simulink model "ev3_robot_hostcontrol_modified"  (R2019b)
settings: Solver=VariableStepAuto  StartTime=0.0  StopTime=inf  RelTol=1e-3
libraries: instrumentlib x4
settings Model: Creator=The MathWorks, Inc.  LastModifiedBy=Duc
settings DataIOCC: ReturnWorkspaceOutputs=off
settings DebuggingCC: ParameterPrecisionLossMsg=none  ArithmeticOperatorsInVariantConditions=warning
settings SFSimCC: SimUseLocalCustomCode=off  CustomCodeUndefinedFunction=UseInterfaceOnly
settings RTWCC: RTWUseLocalCustomCode=off
settings CodeAppCC: StateflowObjectComments=on

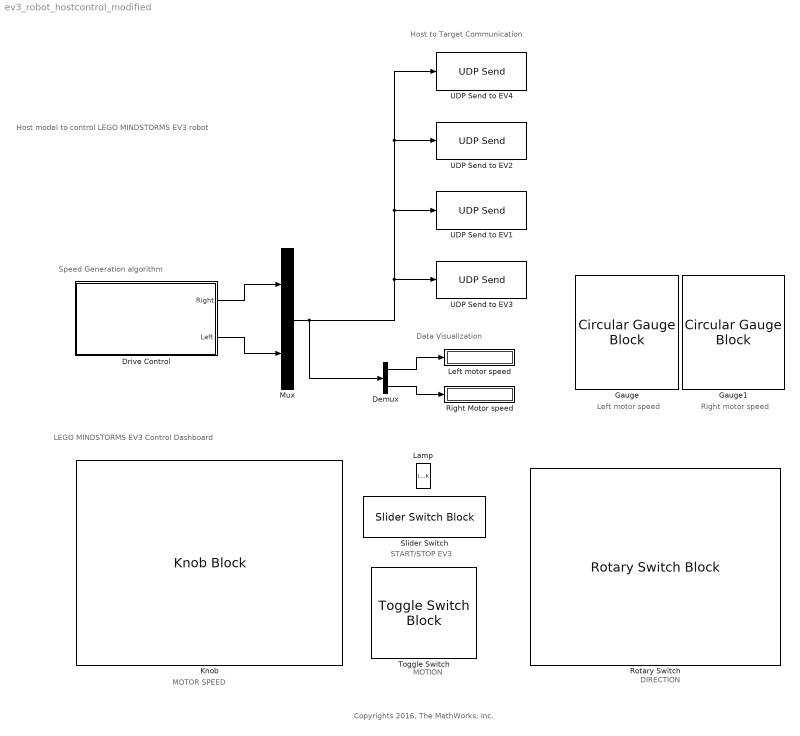
== system ev3_robot_hostcontrol_modified ==
  note: Copyrights 2016, The MathWorks, Inc.
  note: Host model to control
      | LEGO MINDSTORMS EV3 robot
  note: Right motor speed
  note: Left motor speed
  note: DIRECTION
  note: MOTION
  note: START/STOP EV3
  note: MOTOR SPEED
  note: Data Visualization
  note: Host to Target Communication
  note: Speed Generation algorithm
  note: LEGO MINDSTORMS EV3 Control Dashboard
  Demux : Demux  Outputs=2
  Drive Control : Subsystem
  Gauge : CircularGaugeBlock  ScaleMin=-100
  Gauge1 : CircularGaugeBlock  ScaleMin=-100
  Knob : KnobBlock
  Lamp : LampBlock  LabelPosition=Hide
  Left motor speed : Display
  Mux : Mux  Inputs=2
  Right Motor speed : Display
  Rotary Switch : RotarySwitchBlock  LabelPosition=Hide
      settings: Values={{'LEFT', '', 'STRAIGHT', '', 'RIGHT'}, [0 1 2 3 4]}
  Slider Switch : SliderSwitchBlock  LabelPosition=Hide
      settings: Values={{'STOP', 'START'}, [0 1]}
  Toggle Switch : ToggleSwitchBlock  LabelPosition=Hide
      settings: Values={{'REVERSE', 'FORWARD'}, [-1 1]}
  UDP Send to EV1 : instrumentlib/UDP Send  Host=192.168.1.5  Port=25000  LocalPort=-1  EnablePortSharing=off  ByteOrder=LittleEndian  OutputDatagramPacketSize=512  EnableBlockingMode=on  LocalAddress=0.0.0.0
      settings: SourceProductName=Instrument Control Toolbox
  UDP Send to EV2 : instrumentlib/UDP Send  Host=192.168.1.4  Port=25000  LocalPort=-1  EnablePortSharing=off  ByteOrder=LittleEndian  OutputDatagramPacketSize=512  EnableBlockingMode=on  LocalAddress=0.0.0.0
      settings: SourceProductName=Instrument Control Toolbox
  UDP Send to EV3 : instrumentlib/UDP Send  Host=192.168.1.2  Port=25000  LocalPort=-1  EnablePortSharing=off  ByteOrder=LittleEndian  OutputDatagramPacketSize=512  EnableBlockingMode=on  LocalAddress=0.0.0.0
      settings: SourceProductName=Instrument Control Toolbox
  UDP Send to EV4 : instrumentlib/UDP Send  Host=192.168.1.3  Port=25000  LocalPort=-1  EnablePortSharing=off  ByteOrder=LittleEndian  OutputDatagramPacketSize=512  EnableBlockingMode=on  LocalAddress=0.0.0.0
      settings: SourceProductName=Instrument Control Toolbox
  wires:
  Demux/1 -> Left motor speed/1
  Demux/2 -> Right Motor speed/1
  Drive Control/1(Right) -> Mux/1
  Drive Control/2(Left) -> Mux/2
  Mux/1 -> UDP Send to EV2/1, UDP Send to EV4/1, UDP Send to EV1/1, UDP Send to EV3/1, Demux/1

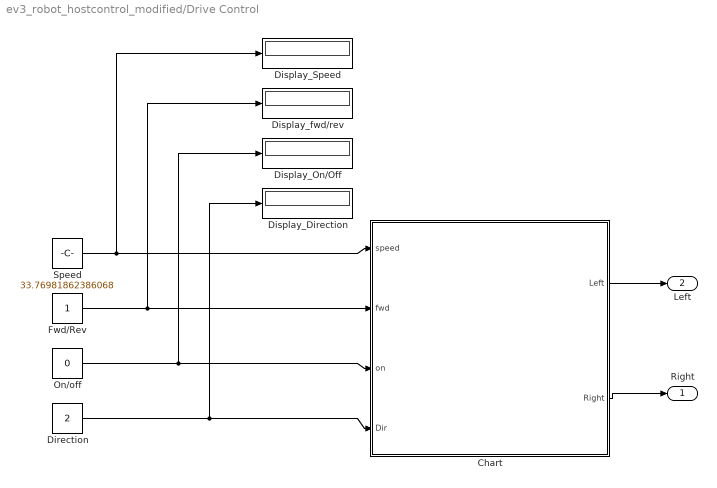
== system ev3_robot_hostcontrol_modified/Drive Control ==
  Chart : Stateflow chart  TreatAsAtomicUnit=on
  Direction : Constant  Value=2  OutDataTypeStr=int8  SampleTime=0.01
  Display_Direction : Display
  Display_On/Off : Display
  Display_Speed : Display
  Display_fwd/rev : Display
  Fwd/Rev : Constant  OutDataTypeStr=int8  SampleTime=0.01
  On/off : Constant  Value=0  OutDataTypeStr=int8  SampleTime=0.01
  Speed : Constant  Value=33.76981862386068  OutDataTypeStr=int8  SampleTime=0.01
  Right : Outport  OutDataTypeStr=int8  PortDimensions=1  VectorParamsAs1DForOutWhenUnconnected=off
  Left : Outport  Port=2  OutDataTypeStr=int8  PortDimensions=1  VectorParamsAs1DForOutWhenUnconnected=off
  wires:
  Chart/2(Right) -> Right/1
  Speed/1 -> Display_Speed/1, Chart/1(speed)
  Direction/1 -> Display_Direction/1, Chart/4(Dir)
  Fwd/Rev/1 -> Display_fwd/rev/1, Chart/2(fwd)
  On/off/1 -> Display_On/Off/1, Chart/3(on)
  Chart/1(Left) -> Left/1

== stateflow chart ev3_robot_hostcontrol_modified/Drive Control/Chart ==
  state Straight
    during:
    Left = speed*fwd*on;
    Right = Left;
  state Left_Diagonal
    during:
    Right = speed*fwd*on;
    Left = 0.5*Right;
  state Right_Diagonal
    during:
    Left = speed*fwd*on;
    Right = 0.5*Left;
  state Right
    during:
    Left = speed*on;
    Right= -1*Left;
  state Left
    during:
    Right = speed*on;
    Left = -1*Right;
  Right_Diagonal -> Left_Diagonal [order 3] : [Dir ==1]
  Left_Diagonal -> Right_Diagonal [order 3] : [Dir ==3]
  (default) -> Straight
  Left -> Straight [order 1] : [Dir ==2]
  Straight -> Left [order 4] : [Dir ==0]
  Straight -> Left_Diagonal [order 1] : [Dir ==1]
  Left_Diagonal -> Straight [order 1] : [Dir ==2]
  Right -> Straight [order 1] : [Dir ==2]
  Straight -> Right [order 3] : [Dir ==4]
  Right_Diagonal -> Straight [order 1] : [Dir ==2]
  Straight -> Right_Diagonal [order 2] : [Dir ==3]
  Left_Diagonal -> Right [order 4] : [Dir ==4]
  Left -> Right_Diagonal [order 4] : [Dir ==3]
  Right -> Left_Diagonal [order 3] : [Dir ==1]
  Right_Diagonal -> Left [order 4] : [Dir ==0]
  Right_Diagonal -> Right [order 2] : [Dir ==4]
  Right -> Right_Diagonal [order 4] : [Dir ==3]
  Left_Diagonal -> Left [order 2] : [Dir ==0]
  Left -> Left_Diagonal [order 2] : [Dir ==1]
  Right -> Left [order 2] : [Dir ==0]
  Left -> Right [order 3] : [Dir ==4]
  data: Left output int8 size=1; speed input; fwd input; on input; Dir input; Right output int8
